simulink model "model"  (R2019b)
settings: Solver=VariableStepAuto  StartTime=0.0  StopTime=10000  RelTol=1e-3  EnableMultiTasking=on
settings Model: Creator=jd33790  LastModifiedBy=jd33790
settings DataIOCC: ReturnWorkspaceOutputs=off
settings OptimizationCC: LifeSpan=inf
settings DebuggingCC: SFUnexpectedBacktrackingDiag=warning  SFNoUnconditionalDefaultTransitionDiag=warning  ArithmeticOperatorsInVariantConditions=warning
settings SFSimCC: SimUseLocalCustomCode=off  CustomCodeUndefinedFunction=UseInterfaceOnly
settings RTWCC: RTWUseLocalCustomCode=off
settings CodeAppCC: StateflowObjectComments=on
settings GRTTargetCC: TargetLangStandard=C89/C90 (ANSI)  GeneratePreprocessorConditionals=Disable all
settings ConfigComp: CovMetricSettings=dw  CovHtmlReporting=on  CovSaveCumulativeToWorkspaceVar=on  CovSaveSingleToWorkspaceVar=on  CovExternalEMLEnable=off

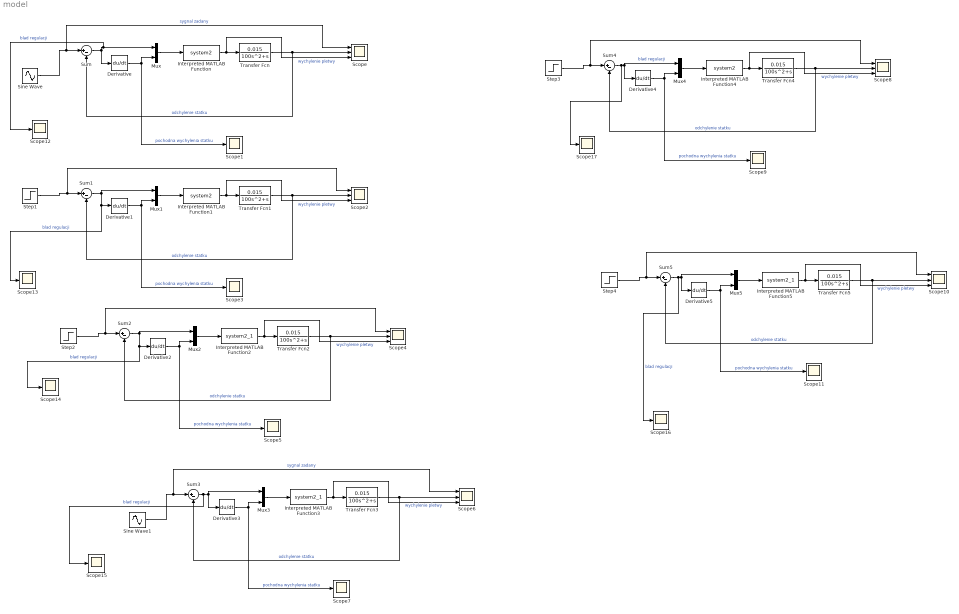
== system model ==
  Derivative{,1..5} (6 alike) : Derivative
  Interpreted MATLAB Function : MATLABFcn  MATLABFcn=system2
  Interpreted MATLAB Function1 : MATLABFcn  MATLABFcn=system2
  Interpreted MATLAB Function2 : MATLABFcn  MATLABFcn=system2_1
  Interpreted MATLAB Function3 : MATLABFcn  MATLABFcn=system2_1
  Interpreted MATLAB Function4 : MATLABFcn  MATLABFcn=system2
  Interpreted MATLAB Function5 : MATLABFcn  MATLABFcn=system2_1
  Mux{,1..5} (6 alike) : Mux  Inputs=2
  Scope{,2,4,6,8,10} (6 alike) : Scope  NumInputPorts=3
  Scope{1,3,5,7,9,11..17} (12 alike) : Scope
  Sine Wave : Sin  Amplitude=20  Frequency=0.001  SampleTime=0
  Sine Wave1 : Sin  Amplitude=20  Frequency=0.001  SampleTime=0
  Step1 : Step  Time=500  After=-90  SampleTime=0
  Step2 : Step  Time=500  After=-90  SampleTime=0
  Step3 : Step  Time=500  After=60  SampleTime=0
  Step4 : Step  Time=500  After=60  SampleTime=0
  Sum{,1..5} (6 alike) : Sum  Inputs=|+-
  Transfer Fcn{,1..5} (6 alike) : TransferFcn  Numerator=[0.015]  Denominator=[100 1 0 ]
  wires:
  Mux/1 -> Interpreted MATLAB Function/1
  Interpreted MATLAB Function/1 -> Scope/3, Transfer Fcn/1  "wychylenie pletwy"
  Transfer Fcn/1 -> Scope/2, Sum/2  "odchylenie statku"
  Derivative/1 -> Mux/2, Scope1/1  "pochodna wychylenia statku"
  Sine Wave/1 -> Scope/1, Sum/1  "sygnal zadany"
  Sum1/1 -> Scope13/1, Derivative1/1, Mux1/1  "blad regulacji"
  Interpreted MATLAB Function1/1 -> Scope2/3, Transfer Fcn1/1  "wychylenie pletwy"
  Transfer Fcn1/1 -> Scope2/2, Sum1/2  "odchylenie statku"
  Derivative1/1 -> Mux1/2, Scope3/1  "pochodna wychylenia statku"
  Mux1/1 -> Interpreted MATLAB Function1/1
  Step1/1 -> Scope2/1, Sum1/1
  Derivative2/1 -> Mux2/2, Scope5/1  "pochodna wychylenia statku"
  Interpreted MATLAB Function2/1 -> Scope4/3, Transfer Fcn2/1  "wychylenie pletwy"
  Mux2/1 -> Interpreted MATLAB Function2/1
  Step2/1 -> Scope4/1, Sum2/1
  Transfer Fcn2/1 -> Scope4/2, Sum2/2  "odchylenie statku"
  Sum2/1 -> Scope14/1, Derivative2/1, Mux2/1  "blad regulacji"
  Sum3/1 -> Scope15/1, Derivative3/1, Mux3/1  "blad regulacji"
  Interpreted MATLAB Function3/1 -> Scope6/3, Transfer Fcn3/1  "wychylenie pletwy"
  Derivative3/1 -> Mux3/2, Scope7/1  "pochodna wychylenia statku"
  Transfer Fcn3/1 -> Scope6/2, Sum3/2  "odchylenie statku"
  Sine Wave1/1 -> Scope6/1, Sum3/1  "sygnal zadany"
  Mux3/1 -> Interpreted MATLAB Function3/1
  Step3/1 -> Scope8/1, Sum4/1
  Interpreted MATLAB Function4/1 -> Scope8/3, Transfer Fcn4/1  "wychylenie pletwy"
  Mux4/1 -> Interpreted MATLAB Function4/1
  Transfer Fcn4/1 -> Scope8/2, Sum4/2  "odchylenie statku"
  Sum4/1 -> Scope17/1, Derivative4/1, Mux4/1  "blad regulacji"
  Derivative4/1 -> Mux4/2, Scope9/1  "pochodna wychylenia statku"
  Sum5/1 -> Scope16/1, Derivative5/1, Mux5/1  "blad regulacji"
  Derivative5/1 -> Mux5/2, Scope11/1  "pochodna wychylenia statku"
  Interpreted MATLAB Function5/1 -> Scope10/3, Transfer Fcn5/1  "wychylenie pletwy"
  Step4/1 -> Scope10/1, Sum5/1
  Transfer Fcn5/1 -> Scope10/2, Sum5/2  "odchylenie statku"
  Mux5/1 -> Interpreted MATLAB Function5/1
  Sum/1 -> Derivative/1, Mux/1, Scope12/1  "blad regulacji"
